simulink model "two_channel_force_force"  (R2022b)
settings: Solver=VariableStepAuto  StartTime=0.0  StopTime=10.0  RelTol=1e-3
values from neighbouring files (symbols this model uses):
  A = 1    [four_channel_bilateral_teleoperation_params.m]
  Be = 100    [four_channel_bilateral_teleoperation_params.m]
  Bh = 1    [four_channel_bilateral_teleoperation_params.m]
  Bm = 20*0.8    (= 16)    [four_channel_bilateral_teleoperation_params.m]
  Bs = 4*Bm    (= 64)    [four_channel_bilateral_teleoperation_params.m]
  Dh = 20*0.8    (= 16)    [four_channel_bilateral_teleoperation_params.m]
  Fc = 0.5    [four_channel_bilateral_teleoperation_params.m]
  Flp = 0.5    [four_channel_bilateral_teleoperation_params.m]
  Jh = 1    [four_channel_bilateral_teleoperation_params.m]
  Ke = 200    [four_channel_bilateral_teleoperation_params.m]
  Km = 10*1    (= 10)    [four_channel_bilateral_teleoperation_params.m]
  Ks = 4*Km    (= 40)    [four_channel_bilateral_teleoperation_params.m]
  Mm = 0.5    [four_channel_bilateral_teleoperation_params.m]
  Ms = 2    [four_channel_bilateral_teleoperation_params.m]
  Ph = 10*1    (= 10)    [four_channel_bilateral_teleoperation_params.m]
  time_delay = 0.1    [four_channel_bilateral_teleoperation_params.m]
  xe = 2    [four_channel_bilateral_teleoperation_params.m]
settings Model: Creator=Manu  LastModifiedBy=Manu

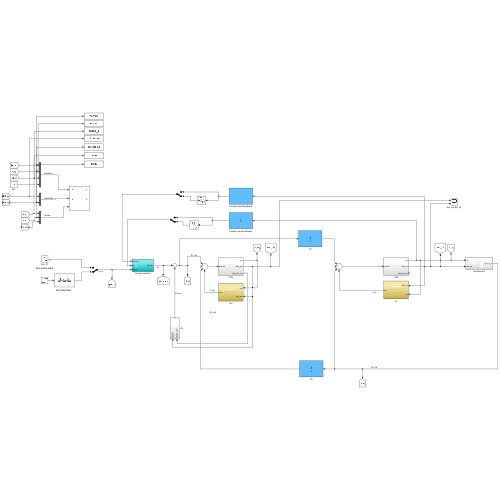
[thumbnail: Simulink's stored preview of the top-level diagram]
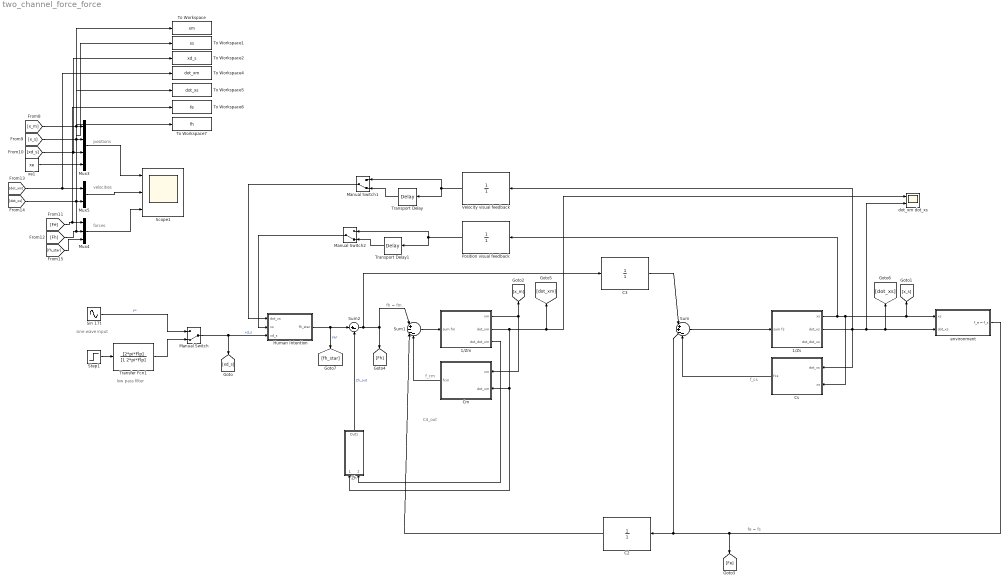
== system two_channel_force_force ==
  note: fe = fs
  note: C4_out
  note: f_cm
  note: fh = fm
  note: sine wave input
  note: low pass filter
  note: f_cs
  note: velocities
  note: positions
  note: forces
  1/Zm : Subsystem
  1/Zs : Subsystem
  C2 : TransferFcn  Denominator=[1]
  C3 : TransferFcn  Denominator=[1]
  Cm : Subsystem
  Cs : Subsystem
  Human Intention : Subsystem
  Manual Switch : ManualSwitch  CurrentSetting=0
  Manual Switch1 : ManualSwitch  CurrentSetting=0
  Manual Switch2 : ManualSwitch  CurrentSetting=0
  Mux3 : Mux
  Mux4 : Mux  Inputs=3
  Mux5 : Mux  Inputs=2
  Position visual feedback : TransferFcn  Denominator=[1]
  Scope1 : Scope  NumInputPorts=3
  Sin 17t : Sin  Amplitude=A  Frequency=2*pi*Fc  SampleTime=0
  Step1 : Step  Time=0.5  After=A  SampleTime=0
  Sum : Sum  Inputs=|++--
  Sum1 : Sum  Inputs=|+---
  Sum2 : Sum  Inputs=|+-
  To Workspace : ToWorkspace  VariableName=xm  SaveFormat=Timeseries  SampleTime=-1
  To Workspace1 : ToWorkspace  VariableName=xs  SaveFormat=Timeseries  SampleTime=-1
  To Workspace2 : ToWorkspace  VariableName=xd_s  SaveFormat=Timeseries  SampleTime=-1
  To Workspace4 : ToWorkspace  VariableName=dot_xm  SaveFormat=Timeseries  SampleTime=-1
  To Workspace5 : ToWorkspace  VariableName=dot_xs  SaveFormat=Timeseries  SampleTime=-1
  To Workspace6 : ToWorkspace  VariableName=fe  SaveFormat=Timeseries  SampleTime=-1
  To Workspace7 : ToWorkspace  VariableName=fh  SaveFormat=Timeseries  SampleTime=-1
  Transfer Fcn1 : TransferFcn  Numerator=[2*pi*Flp]  Denominator=[1 2*pi*Flp]
  Transport Delay : TransportDelay  DelayTime=time_delay
  Transport Delay1 : TransportDelay  DelayTime=time_delay
  Velocity visual feedback : TransferFcn  Denominator=[1]
  Zh : Subsystem
  dot_xm dot_xs : Scope  NumInputPorts=2
  environment : Subsystem
  xe1 : Constant  Value=xe
  wires:
  1/Zm/2(dot_xm) -> dot_xm dot_xs/1, [dot_xm], Cm/2(dot_xm), Zh/1(dot_xm)
  1/Zm/1(xm) -> Cm/1(xm), [x_m]
  Manual Switch/1 -> [xd_s], Human Intention/3(xd_s)  "xd_s"
  Zh/1(Out1) -> Sum2/2  "Zh_out"
  Sin 17t/1 -> Manual Switch/1  "F*"
  1/Zm/3(dot_dot_xm) -> Zh/2(dot_dot_xm)
  Human Intention/1(fh_star) -> Sum2/1, [fh_star]  "fh*"
  Transfer Fcn1/1 -> Manual Switch/2
  Step1/1 -> Transfer Fcn1/1
  Sum2/1 -> C3/1, Sum1/1, [Fh]
  Sum1/1 -> 1/Zm/1(sum fm)
  C3/1 -> Sum/1
  Cs/1(fcs) -> Sum/4
  Sum/1 -> 1/Zs/1(sum fs)
  1/Zs/2(dot_xs) -> Velocity visual feedback/1, Cs/1(dot_xs), dot_xm dot_xs/2, [dot_xs], environment/2(dot_xs)
  1/Zs/1(xs) -> Cs/2(xs), [x_s], environment/1(xs), Position visual feedback/1
  environment/1(f_e = f_s) -> C2/1, Sum/3, [Fe]
  Cm/1(fcm) -> Sum1/4
  C2/1 -> Sum1/3
  Velocity visual feedback/1 -> Transport Delay/1, Manual Switch1/1
  Transport Delay/1 -> Manual Switch1/2
  Manual Switch1/1 -> Human Intention/1(dot_xs)
  Transport Delay1/1 -> Manual Switch2/2
  Position visual feedback/1 -> Transport Delay1/1, Manual Switch2/1
  Manual Switch2/1 -> Human Intention/2(xs)
  Mux3/1 -> Scope1/1
  [dot_xm] -> Mux5/1, To Workspace4/1
  [x_s] -> To Workspace1/1, Mux3/2
  [x_m] -> To Workspace/1, Mux3/1
  [fh_star] -> Mux4/3
  [dot_xs] -> To Workspace5/1, Mux5/2
  Mux5/1 -> Scope1/2
  Mux4/1 -> Scope1/3
  xe1/1 -> Mux3/4
  [Fh] -> To Workspace7/1, Mux4/2
  [Fe] -> Mux4/1, To Workspace6/1
  [xd_s] -> To Workspace2/1, Mux3/3

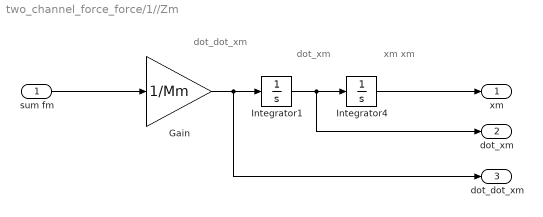
== system two_channel_force_force/1//Zm ==
  note: dot_dot_xm
  note: dot_xm
  note: xm
      | xm
  sum fm : Inport
  Gain : Gain  Gain=1/Mm
  Integrator1 : Integrator
  Integrator4 : Integrator
  xm : Outport
  dot_xm : Outport  Port=2
  dot_dot_xm : Outport  Port=3
  wires:
  sum fm/1 -> Gain/1
  Gain/1 -> dot_dot_xm/1, Integrator1/1
  Integrator4/1 -> xm/1
  Integrator1/1 -> dot_xm/1, Integrator4/1

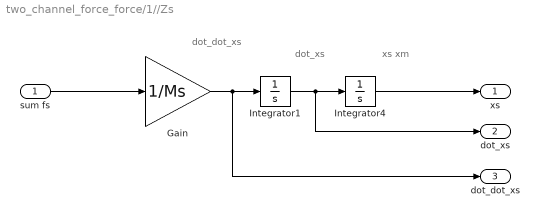
== system two_channel_force_force/1//Zs ==
  note: dot_dot_xs
  note: dot_xs
  note: xs
      | xm
  sum fs : Inport
  Gain : Gain  Gain=1/Ms
  Integrator1 : Integrator
  Integrator4 : Integrator
  xs : Outport
  dot_xs : Outport  Port=2
  dot_dot_xs : Outport  Port=3
  wires:
  sum fs/1 -> Gain/1
  Gain/1 -> dot_dot_xs/1, Integrator1/1
  Integrator4/1 -> xs/1
  Integrator1/1 -> dot_xs/1, Integrator4/1

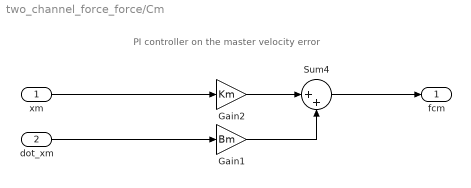
== system two_channel_force_force/Cm ==
  note: PI controller on the master velocity error
  xm : Inport
  dot_xm : Inport  Port=2
  Gain1 : Gain  Gain=Bm
  Gain2 : Gain  Gain=Km
  Sum4 : Sum  Inputs=|++
  fcm : Outport
  wires:
  Sum4/1 -> fcm/1
  xm/1 -> Gain2/1
  Gain2/1 -> Sum4/1
  dot_xm/1 -> Gain1/1
  Gain1/1 -> Sum4/2

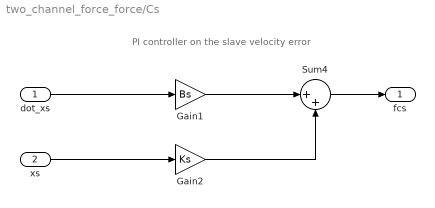
== system two_channel_force_force/Cs ==
  note: PI controller on the slave velocity error
  dot_xs : Inport
  xs : Inport  Port=2
  Gain1 : Gain  Gain=Bs
  Gain2 : Gain  Gain=Ks
  Sum4 : Sum  Inputs=|++
  fcs : Outport
  wires:
  Sum4/1 -> fcs/1
  xs/1 -> Gain2/1
  Gain2/1 -> Sum4/2
  dot_xs/1 -> Gain1/1
  Gain1/1 -> Sum4/1

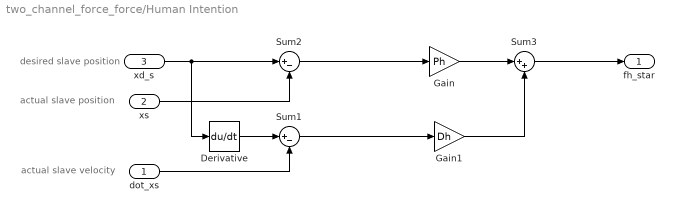
== system two_channel_force_force/Human Intention ==
  note: actual slave velocity
  note: actual slave position
  note: desired slave position
  dot_xs : Inport
  xs : Inport  Port=2
  xd_s : Inport  Port=3
  Derivative : Derivative
  Gain : Gain  Gain=Ph
  Gain1 : Gain  Gain=Dh
  Sum1 : Sum  Inputs=|+-
  Sum2 : Sum  Inputs=|+-
  Sum3 : Sum  Inputs=|++
  fh_star : Outport
  wires:
  xs/1 -> Sum2/2
  dot_xs/1 -> Sum1/2
  Sum2/1 -> Gain/1
  Sum1/1 -> Gain1/1
  Gain1/1 -> Sum3/2
  Gain/1 -> Sum3/1
  Sum3/1 -> fh_star/1
  xd_s/1 -> Derivative/1, Sum2/1
  Derivative/1 -> Sum1/1

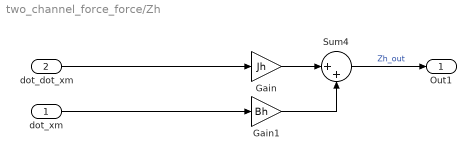
== system two_channel_force_force/Zh ==
  dot_xm : Inport
  dot_dot_xm : Inport  Port=2
  Gain : Gain  Gain=Jh
  Gain1 : Gain  Gain=Bh
  Sum4 : Sum  Inputs=|++
  Out1 : Outport
  wires:
  dot_dot_xm/1 -> Gain/1
  Gain1/1 -> Sum4/2
  Gain/1 -> Sum4/1
  Sum4/1 -> Out1/1  "Zh_out"
  dot_xm/1 -> Gain1/1

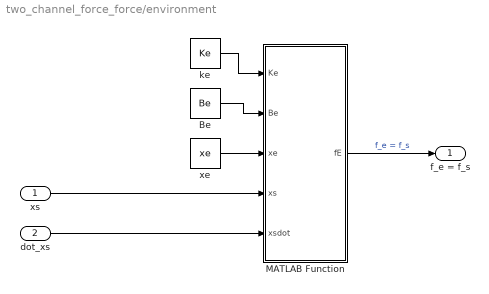
== system two_channel_force_force/environment ==
  xs : Inport
  dot_xs : Inport  Port=2
  Be : Constant  Value=Be
  MATLAB Function : MATLAB Function  TreatAsAtomicUnit=on
  ke : Constant  Value=Ke
  xe : Constant  Value=xe
  f_e = f_s : Outport
  wires:
  MATLAB Function/1(fE) -> f_e = f_s/1  "f_e = f_s"
  xs/1 -> MATLAB Function/4(xs)
  xe/1 -> MATLAB Function/3(xe)
  dot_xs/1 -> MATLAB Function/5(xsdot)
  ke/1 -> MATLAB Function/1(Ke)
  Be/1 -> MATLAB Function/2(Be)

== matlab function two_channel_force_force/environment/MATLAB Function ==
  data: Ke input; fE output; Be input; xe input; xs input; xsdot input
function fE = environment(Ke, Be, xe, xs, xsdot)
    if xs > xe
        fE = Ke * (xs - xe) + Be * xsdot; % Plot both contributions Ke and Be
    else
        fE = 0;
    end
end
